simulink model "PMSM_FOC_Traction"  (R2020b)
settings: Solver=FixedStepAuto  StartTime=0.0  StopTime=10  RelTol=1e-3
model workspace (MAT data in the model file):
  wc : Simulink.Parameter (value not decoded)
values from neighbouring files (symbols this model uses):
  Cosine_table = 1.0 0.99999529 0.99999058 0.99998587 0.99998116 0.99996704 0.99995291 0.99993885 0.99992472 0.99990118 0.99987763 0.99985409 0.9998306 0.99979764 0.99976468 0.99973178 0.99969882 0.99965644 0.99961412 0.99957174 0.99952942 0.99947762 0.99942589 0.99937415 0.99932235 0.9992612 0.99920005 0.99913889 0.99907768 0.99900717 0.99893659 0.99886602 0.99879545 0.99871546 0.99863547 0.99855554 0.99847555 0.    [Hall_HSMO_FOC_Data.sldd]    (also in Hall_SMO_FOC_Data.sldd)
  Flux = 0.0109    [G474_FOC_HSMO.sldd]    (also in Hall_HSMO_FOC_Data.sldd = 0.00529276
  MTPA_id_table = 0.22889 0.23462678 0.23770036 0.2381243 0.23591207 0.23107713 0.2236329 0.21359272 0.20096992 0.18577772 0.16802935 0.14773798 0.12491672 0.099578641 0.071736768 0.041404068 0.0085934745 -0.026682133 -0.064409919 -0.10457709 -0.14717092 -0.1921787 -0.2395878 -0.28938559 -0.34155953 -0.39609709 -0.45298585 -0.51221335 -0.57376724 -0.63763517 -0.70380485 -0.77226412 -0.84300071 -0.91600245 -0.991257    [Hall_HSMO_FOC_Data.sldd]    (also in Hall_SMO_FOC_Data.sldd)
  MTPA_iq_table = -1.0417 -0.16083497 0.71926296 1.5985928 2.4771533 3.3549435 4.2319627 5.1082091 5.9836826 6.8583813 7.732305 8.6054525 9.4778223 10.349415 11.220228 12.090261 12.959513 13.827983 14.69567 15.562573 16.428694 17.294027 18.158575 19.022335 19.885307 20.747492 21.608887 22.469492 23.329306 24.188328 25.046556 25.903992 26.760633 27.616482 28.471533 29.325788 30.179247 31.031908 31.883772 32.734837 3    [Hall_HSMO_FOC_Data.sldd]    (also in Hall_SMO_FOC_Data.sldd)
  MTPA_Te_Max = 800.0    [Hall_HSMO_FOC_Data.sldd]    (also in Hall_SMO_FOC_Data.sldd)
  MTPA_Te_Min = 0.0    [Hall_HSMO_FOC_Data.sldd]    (also in Hall_SMO_FOC_Data.sldd)
  Sine_table = 0.0 0.0015339879 0.0030679768 0.0046019657 0.0061359555 0.0076698866 0.0092038177 0.010737749 0.012271681 0.013805497 0.015339312 0.016873131 0.018406944 0.019940587 0.021474229 0.023007872 0.024541514 0.026074925 0.027608337 0.029141748 0.03067516 0.032208283 0.033741407 0.035274528 0.036807653 0.038340431 0.039873205 0.04140598 0.042938754 0.04447113 0.046003502 0.047535874 0.049068246 0.0506001    [Hall_HSMO_FOC_Data.sldd]    (also in Hall_SMO_FOC_Data.sldd)
undefined symbols (not defined in the file or in its folder): CL_Param, ctrlParamsPI, DiscIntNeverNeededParam, Flux_weak, FluxObsever, Hall_Parameter, HFI, inverter, Kiv, Kiw, Kpv, Kpw, magnitude, OPL_Param, pmsm, Resolver_Parameter, sigbuilder_block, SMO, SVPWM, Vdc
libraries: powerlib x29, fl_lib x18, simulink x7, nesl_utility x7, pid_lib x5, dspstat3 x4, eeGeneralControl x4, eeDiscretePi x2, powerlib_extras x1, ee_lib x1
(part 5 of 6)

== system PMSM_FOC_Traction/Motor_Control/Motor_Control_Funtion/Control_Command_2ms/Speed_PI/Speed_PI/Speed_Control ==
  Err : Inport
  Action Port : ActionPort  ActionPortLabel=if((u1==3)&(u2==1))
  Add : Sum
  Cons : Constant  Value=0  OutDataTypeStr=single
  Discrete-Time Integrator : DiscreteIntegrator  SampleTime=-1  ICPrevOutput=DiscIntNeverNeededParam  ICPrevScaledInput=DiscIntNeverNeededParam
  Ki : Constant  Value=ctrlParamsPI.speed_PI_Ki  OutDataTypeStr=single
  Kp : Constant  Value=ctrlParamsPI.speed_PI_Kp  OutDataTypeStr=single
  Product : Product
  Product1 : Product
  Relational Operator1 : RelationalOperator  Operator===  OutDataTypeStr=boolean  RndMeth=Simplest
  Saturation : Saturate  UpperLimit=ctrlParamsPI.speed_PI_OutputMax  LowerLimit=ctrlParamsPI.speed_PI_OutputMin
  Scope : Scope
  Switch : Switch  Criteria=u2 > Threshold
  Unit Delay3 : UnitDelay  SampleTime=-1  HasFrameUpgradeWarning=on
  PI_Out : Outport
  wires:
  Kp/1 -> Product/1
  Err/1 -> Switch/1, Product/2
  Switch/1 -> Product1/2
  Product1/1 -> Discrete-Time Integrator/1
  Product/1 -> Add/1
  Add/1 -> Relational Operator1/1, Saturation/1
  Saturation/1 -> Relational Operator1/2, PI_Out/1
  Discrete-Time Integrator/1 -> Add/2, Scope/1
  Relational Operator1/1 -> Unit Delay3/1
  Ki/1 -> Product1/1
  Unit Delay3/1 -> Switch/2
  Cons/1 -> Switch/3

== system PMSM_FOC_Traction/Motor_Control/Motor_Control_Funtion/Control_Command_2ms/Speed_PI/Speed_PI/Speed_Control1 ==
  Err : Inport
  Action Port : ActionPort  ActionPortLabel=elseif((u2==0) & ((u3~=2)&(u3~=3)))
  Add : Sum
  Cons : Constant  Value=0  OutDataTypeStr=single
  Discrete-Time Integrator : DiscreteIntegrator  SampleTime=-1  ICPrevOutput=DiscIntNeverNeededParam  ICPrevScaledInput=DiscIntNeverNeededParam
  Ki : Constant  Value=ctrlParamsPI.speed_PI_Ki  OutDataTypeStr=single
  Kp : Constant  Value=ctrlParamsPI.speed_PI_Kp  OutDataTypeStr=single
  Product : Product
  Product1 : Product
  Relational Operator1 : RelationalOperator  Operator===  OutDataTypeStr=boolean  RndMeth=Simplest
  Saturation : Saturate  UpperLimit=ctrlParamsPI.speed_PI_OutputMax  LowerLimit=ctrlParamsPI.speed_PI_OutputMin
  Switch : Switch  Criteria=u2 > Threshold
  Unit Delay3 : UnitDelay  SampleTime=-1  HasFrameUpgradeWarning=on
  PI_Out : Outport
  wires:
  Kp/1 -> Product/1
  Err/1 -> Switch/1, Product/2
  Switch/1 -> Product1/2
  Product1/1 -> Discrete-Time Integrator/1
  Product/1 -> Add/1
  Add/1 -> Relational Operator1/1, Saturation/1
  Saturation/1 -> Relational Operator1/2, PI_Out/1
  Discrete-Time Integrator/1 -> Add/2
  Relational Operator1/1 -> Unit Delay3/1
  Ki/1 -> Product1/1
  Unit Delay3/1 -> Switch/2
  Cons/1 -> Switch/3

== system PMSM_FOC_Traction/Motor_Control/Motor_Control_Funtion/FOC_Control_100us/FOC/Angle_set/Subsystem ==
  HFI_state : Inport
  HFI_angle : Inport  Port=2
  IPD_Angle : Inport  Port=3
  Action Port : ActionPort  ActionPortLabel=if(u1 ==1)
  If1 : If  IfExpression=u1 ==3  ElseIfExpressions=u1 <3  ShowElse=off
  Merge : Merge
  Subsystem1 : Subsystem
  Subsystem2 : Subsystem
  Out1 : Outport
  wires:
  HFI_state/1 -> If1/1
  HFI_angle/1 -> Subsystem1/1(HFI_Angle)
  If1/2 -> Subsystem2/Action
  If1/1 -> Subsystem1/Action
  IPD_Angle/1 -> Subsystem2/1(IPD_Angle)
  Merge/1 -> Out1/1
  Subsystem1/1(Out1) -> Merge/1
  Subsystem2/1(Out1) -> Merge/2

== system PMSM_FOC_Traction/Motor_Control/Motor_Control_Funtion/FOC_Control_100us/FOC/Angle_set/Subsystem1 ==
  Reso_angle : Inport
  Action Port : ActionPort  ActionPortLabel=else
  Out1 : Outport
  wires:
  Reso_angle/1 -> Out1/1

== system PMSM_FOC_Traction/Motor_Control/Motor_Control_Funtion/FOC_Control_100us/FOC/Clarke_Transform/Clark1 ==
  Iabc : Inport
  Add : Sum  Inputs=+--
  Add1 : Sum  Inputs=+-
  Demux : Demux  Outputs=3
  Gain : Gain  Gain=0.5
  Gain1 : Gain  Gain=0.5
  Gain2 : Gain  Gain=sqrt(2/3)
  Gain3 : Gain  Gain=sqrt(3)/2
  Gain4 : Gain  Gain=sqrt(3)/2
  Gain5 : Gain  Gain=sqrt(2/3)
  Ialpha : Outport  VectorParamsAs1DForOutWhenUnconnected=off
  Ibeta : Outport  Port=2  VectorParamsAs1DForOutWhenUnconnected=off
  wires:
  Iabc/1 -> Demux/1
  Demux/1 -> Add/1
  Gain/1 -> Add/2
  Demux/2 -> Gain3/1, Gain/1
  Gain1/1 -> Add/3
  Demux/3 -> Gain4/1, Gain1/1
  Add/1 -> Gain2/1
  Gain2/1 -> Ialpha/1
  Gain3/1 -> Add1/1
  Gain4/1 -> Add1/2
  Add1/1 -> Gain5/1
  Gain5/1 -> Ibeta/1

== system PMSM_FOC_Traction/Motor_Control/Motor_Control_Funtion/FOC_Control_100us/FOC/D_Current_PI/ID_Control ==
  Err : Inport
  Add : Sum
  Cons : Constant  Value=0  OutDataTypeStr=single
  Discrete-Time Integrator : DiscreteIntegrator  SampleTime=-1  ICPrevOutput=DiscIntNeverNeededParam  ICPrevScaledInput=DiscIntNeverNeededParam
  Ki : Constant  Value=ctrlParamsPI.ID_Current_PI_Ki  OutDataTypeStr=single
  Kp : Constant  Value=ctrlParamsPI.ID_Current_PI_Kp  OutDataTypeStr=single
  Product : Product
  Product1 : Product
  Relational Operator1 : RelationalOperator  Operator===  OutDataTypeStr=boolean  RndMeth=Simplest
  Saturation : Saturate  UpperLimit=ctrlParamsPI.ID_Current_PI_OutputMax  LowerLimit=ctrlParamsPI.ID_Current_PI_OutputMin
  Switch : Switch  Criteria=u2 > Threshold
  Unit Delay3 : UnitDelay  SampleTime=-1  HasFrameUpgradeWarning=on
  PI_Out : Outport
  wires:
  Kp/1 -> Product/1
  Err/1 -> Switch/1, Product/2
  Switch/1 -> Product1/2
  Product1/1 -> Discrete-Time Integrator/1
  Product/1 -> Add/1
  Add/1 -> Relational Operator1/1, Saturation/1
  Saturation/1 -> Relational Operator1/2, PI_Out/1
  Cons/1 -> Switch/3
  Discrete-Time Integrator/1 -> Add/2
  Relational Operator1/1 -> Unit Delay3/1
  Ki/1 -> Product1/1
  Unit Delay3/1 -> Switch/2

== system PMSM_FOC_Traction/Motor_Control/Motor_Control_Funtion/FOC_Control_100us/FOC/Flux_weakening /Subsystem ==
  Vd : Inport
  Vq : Inport  Port=2
  Id : Inport  Port=3
  Iq : Inport  Port=4
  Action Port : ActionPort  ActionPortLabel=if(u1 ==1)
  Flux_weak : Subsystem  TreatAsAtomicUnit=on  mask{kp=Flux_weak.Kp, ki=Flux_weak.Ki, Id_max=Flux_weak.Idref_max, Id_min=Flux_weak.Idref_min}
      settings: RTWSystemCode=Nonreusable function  RTWFcnNameOpts=Use subsystem name
  Id_ref : Outport
  Iq_ref : Outport  Port=2
  wires:
  Vd/1 -> Flux_weak/1(Vd)
  Vq/1 -> Flux_weak/2(Vq)
  Id/1 -> Flux_weak/3(id_input)
  Iq/1 -> Flux_weak/4(Iq_input)
  Flux_weak/1(Id_ref) -> Id_ref/1
  Flux_weak/2(iq_ref) -> Iq_ref/1

== system PMSM_FOC_Traction/Motor_Control/Motor_Control_Funtion/FOC_Control_100us/FOC/Flux_weakening /Subsystem1 ==
  Id : Inport
  Iq : Inport  Port=2
  Action Port : ActionPort  ActionPortLabel=else
  Id_ref : Outport
  Iq_ref : Outport  Port=2
  wires:
  Id/1 -> Id_ref/1
  Iq/1 -> Iq_ref/1

== system PMSM_FOC_Traction/Motor_Control/Motor_Control_Funtion/FOC_Control_100us/FOC/HF_Observer/HFI_Function ==
  Ialpha-beta : Inport
  Phase_CurrentABC : Inport  Port=2  PortDimensions=3
  Id : Inport  Port=3
  Action Port : ActionPort  ActionPortLabel=if(u1==1)
  Delay : Delay  DelayLength=1  InitialCondition=0
  Delay1 : Delay  DelayLength=1  InitialCondition=0
  Delay2 : Delay  DelayLength=1  InitialCondition=0
  HFI : Subsystem
  HFI_Enalble : Constant  Value=HFI.Func_Enable  OutDataTypeStr=uint8
  HFI_State_machine : Stateflow chart  TreatAsAtomicUnit=on
      settings: RTWSystemCode=Nonreusable function  RTWFcnNameOpts=Use subsystem name
  IPD : Subsystem  TreatAsAtomicUnit=on
      settings: RTWSystemCode=Nonreusable function
  Merge : Merge
  Merge1 : Merge
  Merge2 : Merge
  NS : Subsystem  TreatAsAtomicUnit=on
      settings: RTWSystemCode=Nonreusable function
  Switch Case1 : SwitchCase  CaseConditions={1,2,3}
  RUN_State : Outport
  HFI_State : Outport  Port=2
  HFI_signal : Outport  Port=3
  speed_est : Outport  Port=4
  theta_est : Outport  Port=5
  Ualpha : Outport  Port=6
  Ubeta : Outport  Port=7
  IPD_Theta : Outport  Port=8
  wires:
  NS/1(Ualpha) -> Merge/2
  HFI_State_machine/1(HFI_state) -> HFI_State/1, Switch Case1/1
  Delay/1 -> NS/1(Id)
  Switch Case1/2 -> [NS]
  Id/1 -> Delay/1
  IPD/2(Ubeta) -> Merge1/1
  [NS] -> NS/Action
  HFI/5(theta_est) -> Merge2/2
  IPD/3(Theta) -> Delay1/1
  Phase_CurrentABC/1 -> IPD/1(Iabc)  "Phase_CurrentABC"
  Delay1/1 -> NS/2(Theta)
  HFI/2(speed_est) -> speed_est/1
  Ialpha-beta/1 -> HFI/1(Ialpha-beta)
  Merge1/1 -> Ubeta/1
  Switch Case1/4 -> [default]
  [IPD] -> IPD/Action
  Merge/1 -> Ualpha/1
  [RUN] -> HFI/Action
  NS/2(Ubeta) -> Merge1/2
  Switch Case1/1 -> [IPD]
  HFI_Enalble/1 -> HFI_State_machine/1(HFI_flag)
  HFI/1(HFI_signal) -> HFI_signal/1
  IPD/1(Ualpha) -> Merge/1
  NS/3(IPD_Angle) -> Merge2/1
  Merge2/1 -> theta_est/1
  Switch Case1/3 -> [RUN]
  NS/4(Angle_RUN) -> Delay2/1
  Delay2/1 -> HFI/2(IPD_angle)
  HFI/3(HFI_State) -> RUN_State/1
  HFI/4(IPD_Theta) -> IPD_Theta/1

== system PMSM_FOC_Traction/Motor_Control/Motor_Control_Funtion/FOC_Control_100us/FOC/Q_Current_PI/IQ_Control ==
  Err : Inport
  Add : Sum
  Cons : Constant  Value=0  OutDataTypeStr=single
  Discrete-Time Integrator : DiscreteIntegrator  SampleTime=-1  ICPrevOutput=DiscIntNeverNeededParam  ICPrevScaledInput=DiscIntNeverNeededParam
  Ki : Constant  Value=ctrlParamsPI.IQ_Current_PI_Ki  OutDataTypeStr=single
  Kp : Constant  Value=ctrlParamsPI.IQ_Current_PI_Kp  OutDataTypeStr=single
  Product : Product
  Product1 : Product
  Relational Operator1 : RelationalOperator  Operator===  OutDataTypeStr=boolean  RndMeth=Simplest
  Saturation : Saturate  UpperLimit=ctrlParamsPI.IQ_Current_PI_OutputMax  LowerLimit=ctrlParamsPI.IQ_Current_PI_OutputMin
  Switch : Switch  Criteria=u2 > Threshold
  Unit Delay3 : UnitDelay  SampleTime=-1  HasFrameUpgradeWarning=on
  PI_Out : Outport
  wires:
  Kp/1 -> Product/1
  Err/1 -> Switch/1, Product/2
  Switch/1 -> Product1/2
  Product1/1 -> Discrete-Time Integrator/1
  Product/1 -> Add/1
  Add/1 -> Relational Operator1/1, Saturation/1
  Saturation/1 -> Relational Operator1/2, PI_Out/1
  Cons/1 -> Switch/3
  Discrete-Time Integrator/1 -> Add/2
  Relational Operator1/1 -> Unit Delay3/1
  Ki/1 -> Product1/1
  Unit Delay3/1 -> Switch/2

== system PMSM_FOC_Traction/Motor_Control/Motor_Control_Funtion/FOC_Control_100us/FOC/SVPWM/N Sector  Caculate ==
  Ubelta : Inport
  Ualf : Inport  Port=2
  Add : Sum  Inputs=+++
  Add1 : Sum  Inputs=-+
  Add2 : Sum  Inputs=--
  Constant : Constant  OutDataTypeStr=single
  Constant1 : Constant  Value=0  OutDataTypeStr=single
  Gain : Gain  Gain=sqrt(3)
  Gain1 : Gain  Gain=2
  Gain2 : Gain  Gain=4
  Saturation : Saturate  UpperLimit=6  LowerLimit=1
  Switch : Switch
  Switch1 : Switch
  Switch2 : Switch
  N : Outport
  wires:
  Saturation/1 -> N/1
  Add/1 -> Saturation/1
  Gain2/1 -> Add/3
  Switch2/1 -> Gain2/1
  Add2/1 -> Switch2/2
  Gain1/1 -> Add/2
  Switch1/1 -> Gain1/1
  Add1/1 -> Switch1/2
  Gain/1 -> Add2/2, Add1/2
  Ualf/1 -> Gain/1
  Switch/1 -> Add/1
  Constant1/1 -> Switch/3, Switch1/3, Switch2/3
  Constant/1 -> Switch/1, Switch1/1, Switch2/1
  Ubelta/1 -> Add2/1, Add1/1, Switch/2

== system PMSM_FOC_Traction/Motor_Control/Motor_Control_Funtion/FOC_Control_100us/FOC/SVPWM/T1 T2  Caculate ==
  note: Z
  note: Y
  note: -X
  note: X
  note: -Y
  note: Y
  note: -X
  note: X
  note: Z
  note: -Y
  note: -Z
  note: X
  note: Y
  note: Z
  N : Inport
  X : Inport  Port=2
  Y : Inport  Port=3
  Z : Inport  Port=4
  Tpwm : Inport  Port=5
  Add : Sum
  Add1 : Sum  Inputs=-+
  Divide : Product  Inputs=**/
  Divide1 : Product  Inputs=/**
  Gain : Gain  Gain=-1
  Gain1 : Gain  Gain=-1
  Gain2 : Gain  Gain=-1
  Index Vector : MultiPortSwitch  Inputs=6
  Index Vector1 : MultiPortSwitch  Inputs=6
  Switch : Switch  Criteria=u2 > Threshold
  Switch2 : Switch  Criteria=u2 > Threshold
  T1 : Outport
  T2 : Outport  Port=2
  wires:
  Switch2/1 -> T2/1
  Divide1/1 -> Switch2/3
  Switch/1 -> T1/1
  Add1/1 -> Switch/2, Switch2/2
  Add/1 -> Divide1/1, Divide/3, Add1/1
  Tpwm/1 -> Divide1/2, Divide/2, Add1/2
  Divide/1 -> Switch/3
  Index Vector1/1 -> Switch2/1, Add/2, Divide1/3
  Index Vector/1 -> Switch/1, Divide/1, Add/1
  Gain1/1 -> Index Vector/7, Index Vector1/6
  Gain2/1 -> Index Vector/4, Index Vector1/7  "-Z"
  Gain/1 -> Index Vector/5, Index Vector1/3
  Y/1 -> Gain1/1, Index Vector/3, Index Vector1/2
  X/1 -> Index Vector1/4, Index Vector/6, Gain/1
  Z/1 -> Index Vector/2, Index Vector1/5, Gain2/1
  N/1 -> Index Vector1/1, Index Vector/1

== system PMSM_FOC_Traction/Motor_Control/Motor_Control_Funtion/FOC_Control_100us/FOC/SVPWM/Tcm calculate ==
  note: Tc
  note: Tb
  note: Ta
  N : Inport
  T1 : Inport  Port=2
  T2 : Inport  Port=3
  Tpwm : Inport  Port=4
  Add : Sum  Inputs=--+
  Add1 : Sum
  Add2 : Sum
  Gain : Gain  Gain=0.5
  Gain1 : Gain  Gain=0.5
  Gain2 : Gain  Gain=1/4
  Index Vector : MultiPortSwitch  Inputs=6
  Index Vector1 : MultiPortSwitch  Inputs=6
  Index Vector2 : MultiPortSwitch  Inputs=6
  Scope2 : Scope  NumInputPorts=3
  Tcm1 : Outport
  Tcm2 : Outport  Port=2
  Tcm3 : Outport  Port=3
  wires:
  Index Vector2/1 -> Scope2/3, Tcm3/1
  N/1 -> Index Vector/1, Index Vector1/1, Index Vector2/1
  Add2/1 -> Index Vector/5, Index Vector/6, Index Vector1/3, Index Vector1/7, Index Vector2/2, Index Vector2/4
  Gain1/1 -> Add2/1
  Add1/1 -> Add2/2, Index Vector/2, Index Vector/7, Index Vector1/4, Index Vector1/5, Index Vector2/3, Index Vector2/6
  Gain2/1 -> Index Vector2/5, Index Vector2/7, Add1/2, Index Vector/3, Index Vector/4, Index Vector1/2, Index Vector1/6
  Gain/1 -> Add1/1
  Add/1 -> Gain2/1
  Tpwm/1 -> Add/3
  T2/1 -> Add/2, Gain1/1
  T1/1 -> Add/1, Gain/1
  Index Vector/1 -> Scope2/1, Tcm1/1
  Index Vector1/1 -> Scope2/2, Tcm2/1

== system PMSM_FOC_Traction/Motor_Control/Motor_Control_Funtion/FOC_Control_100us/FOC/SVPWM/XYZ Caculate ==
  note: X
  note: Y
  note: Z
  Ualfpa : Inport
  Ubelta : Inport  Port=2
  Udc : Inport  Port=3
  Tpwm : Inport  Port=4
  Add1 : Sum  Inputs=-+
  Add2 : Sum  Inputs=--
  Constant : Constant  Value=sqrt(3)  OutDataTypeStr=single
  Divide : Product  Inputs=**/
  Gain : Gain  Gain=sqrt(3)
  Gain1 : Gain  Gain=-0.5
  Gain2 : Gain  Gain=-0.5
  Product : Product
  Product1 : Product
  Product2 : Product
  X : Outport
  Y : Outport  Port=2
  Z : Outport  Port=3
  wires:
  Gain2/1 -> Product1/1
  Add2/1 -> Gain2/1
  Add1/1 -> Gain1/1
  Gain/1 -> Add2/2, Add1/2
  Ualfpa/1 -> Gain/1
  Ubelta/1 -> Add2/1, Add1/1, Product/1
  Gain1/1 -> Product2/2
  Product2/1 -> Z/1
  Divide/1 -> Product1/2, Product2/1, Product/2
  Product1/1 -> Y/1
  Product/1 -> X/1
  Udc/1 -> Divide/3
  Tpwm/1 -> Divide/2
  Constant/1 -> Divide/1

== system PMSM_FOC_Traction/Motor_Control/Motor_Control_Funtion/FOC_Control_100us/FOC/Set_Idq/Set_Idq ==
  Id_Command : Inport
  Iq_Command : Inport  Port=2
  Action Port : ActionPort  ActionPortLabel=if(u1==2 | u1==1)
  Id : Outport  VectorParamsAs1DForOutWhenUnconnected=off
  Iq : Outport  Port=2  VectorParamsAs1DForOutWhenUnconnected=off
  wires:
  Id_Command/1 -> Id/1
  Iq_Command/1 -> Iq/1

== system PMSM_FOC_Traction/Motor_Control/Motor_Control_Funtion/FOC_Control_100us/FOC/Set_Idq/Set_Idq1 ==
  Id_Command : Inport
  Iq_Command : Inport  Port=2
  Action Port : ActionPort  ActionPortLabel=else
  Id : Outport  VectorParamsAs1DForOutWhenUnconnected=off
  Iq : Outport  Port=2  VectorParamsAs1DForOutWhenUnconnected=off
  wires:
  Id_Command/1 -> Id/1
  Iq_Command/1 -> Iq/1

== system PMSM_FOC_Traction/Motor_Control/Motor_Control_Funtion/FOC_Control_100us/FOC/Subsystem1/If Action Subsystem1 ==
  In1 : Inport
  In2 : Inport  Port=2
  Action Port : ActionPort  ActionPortLabel=else
  Out1 : Outport
  Out2 : Outport  Port=2
  wires:
  In1/1 -> Out1/1
  In2/1 -> Out2/1

== system PMSM_FOC_Traction/Motor_Control/Motor_Control_Funtion/FOC_Control_100us/FOC/Subsystem1/If Action Subsystem2 ==
  In1 : Inport
  In2 : Inport  Port=2
  Action Port : ActionPort  ActionPortLabel=if((u1<3)&(u1>0))
  Out1 : Outport
  Out2 : Outport  Port=2
  wires:
  In1/1 -> Out1/1
  In2/1 -> Out2/1

== system PMSM_FOC_Traction/Motor_Control/Motor_Control_Funtion/Angle_Speed_100us/Flux_OBSERVER/equ3.12/integrator/RangeLimit ==
  In : Inport  OutDataTypeStr=single
  Constant : Constant  Value=2*pi  OutDataTypeStr=single  SampleTime=-1
  Constant1 : Constant  Value=0  OutDataTypeStr=single  SampleTime=-1
  If : If  NumInputs=2  IfExpression=u1  ElseIfExpressions=u2
  If Action Subsystem : Subsystem  TreatAsAtomicUnit=on
  If Action Subsystem1 : Subsystem  TreatAsAtomicUnit=on
  If Action Subsystem2 : Subsystem  TreatAsAtomicUnit=on
  Merge : Merge  Inputs=3
  Relational Operator : RelationalOperator  Operator=>  OutDataTypeStr=boolean  RndMeth=Simplest
  Relational Operator1 : RelationalOperator  Operator=<  OutDataTypeStr=boolean  RndMeth=Simplest
  Theta : Outport  OutDataTypeStr=single
  wires:
  Relational Operator/1 -> If/1
  Constant/1 -> Relational Operator/2
  Constant1/1 -> Relational Operator1/2
  In/1 -> Relational Operator1/1, If Action Subsystem2/1(In1), If Action Subsystem1/1(In1), If Action Subsystem/1(In1), Relational Operator/1
  Relational Operator1/1 -> If/2
  Merge/1 -> Theta/1
  If/3 -> If Action Subsystem2/Action
  If/2 -> If Action Subsystem/Action
  If/1 -> If Action Subsystem1/Action
  If Action Subsystem2/1(Out1) -> Merge/1
  If Action Subsystem/1(Out1) -> Merge/2
  If Action Subsystem1/1(Out1) -> Merge/3

== system PMSM_FOC_Traction/Motor_Control/Motor_Control_Funtion/Angle_Speed_100us/HIGH_SMO/QPLL/SpeedToTheta/RangeLimit ==
  In : Inport
  Constant : Constant  Value=2*pi  OutDataTypeStr=single  SampleTime=-1
  Constant1 : Constant  Value=0  OutDataTypeStr=single  SampleTime=-1
  If : If  NumInputs=2  IfExpression=u1  ElseIfExpressions=u2
  If Action Subsystem : Subsystem  TreatAsAtomicUnit=on
  If Action Subsystem1 : Subsystem  TreatAsAtomicUnit=on
  If Action Subsystem2 : Subsystem  TreatAsAtomicUnit=on
  Merge : Merge  Inputs=3
  Relational Operator : RelationalOperator  Operator=>  OutDataTypeStr=boolean  RndMeth=Simplest
  Relational Operator1 : RelationalOperator  Operator=<  OutDataTypeStr=boolean  RndMeth=Simplest
  Theta : Outport
  wires:
  Relational Operator/1 -> If/1
  Constant/1 -> Relational Operator/2
  Constant1/1 -> Relational Operator1/2
  In/1 -> Relational Operator1/1, If Action Subsystem2/1(In1), If Action Subsystem1/1(In1), If Action Subsystem/1(In1), Relational Operator/1
  Relational Operator1/1 -> If/2
  Merge/1 -> Theta/1
  If/3 -> If Action Subsystem2/Action
  If/2 -> If Action Subsystem/Action
  If/1 -> If Action Subsystem1/Action
  If Action Subsystem2/1(Out1) -> Merge/1
  If Action Subsystem/1(Out1) -> Merge/2
  If Action Subsystem1/1(Out1) -> Merge/3

== system PMSM_FOC_Traction/Motor_Control/Motor_Control_Funtion/Angle_Speed_100us/HIGH_SMO/QPLL/Subsystem1/If Action Subsystem ==
  Action Port : ActionPort  ActionPortLabel=if(u1 > 0)
  Constant : Constant  OutDataTypeStr=single
  Out1 : Outport
  wires:
  Constant/1 -> Out1/1

== system PMSM_FOC_Traction/Motor_Control/Motor_Control_Funtion/Angle_Speed_100us/HIGH_SMO/QPLL/Subsystem1/If Action Subsystem1 ==
  Action Port : ActionPort  ActionPortLabel=else
  Constant : Constant  Value=-1  OutDataTypeStr=single
  Out1 : Outport
  wires:
  Constant/1 -> Out1/1

== system PMSM_FOC_Traction/Motor_Control/Motor_Control_Funtion/Angle_Speed_100us/SpeedAndAngle/ACC_OMG/BLDC/Control ==
  RPMReq : Inport
  w_sens : Inport  Port=2
  Hall : Inport  Port=3
  BLDC_State : Inport  Port=4
  Commutation : Subsystem
  If1 : If  IfExpression=u1==3  ShowElse=off
  Scope3 : Scope
  Speed_Control : Subsystem
  Sum : Sum  Inputs=|+-
  rad/s->rpm : Gain  Gain=30/pi
  Gate : Outport  VectorParamsAs1DForOutWhenUnconnected=off
  Duty : Outport  Port=2  VectorParamsAs1DForOutWhenUnconnected=off
  wires:
  RPMReq/1 -> Sum/1
  w_sens/1 -> rad/s->rpm/1
  rad/s->rpm/1 -> Sum/2, Scope3/1
  Commutation/1(S) -> Gate/1
  Hall/1 -> Commutation/1(Hall)
  Sum/1 -> Speed_Control/1(Err)
  Speed_Control/1(PI_Out) -> Duty/1
  BLDC_State/1 -> If1/1
  If1/1 -> Speed_Control/Action

== system PMSM_FOC_Traction/Motor_Control/Motor_Control_Funtion/Angle_Speed_100us/SpeedAndAngle/ACC_OMG/Six_point/Sector_1 ==
  Action Port : ActionPort  ActionPortLabel=case [ 1 ]:
  Add : Sum
  Constant : Constant  Value=Hall_Parameter.Sector_1  OutDataTypeStr=single
  Constant1 : Constant  Value=Hall_Parameter.shift  OutDataTypeStr=single
  Angle_0 : Outport
  wires:
  Constant/1 -> Add/1
  Constant1/1 -> Add/2
  Add/1 -> Angle_0/1

== system PMSM_FOC_Traction/Motor_Control/Motor_Control_Funtion/Angle_Speed_100us/SpeedAndAngle/ACC_OMG/Six_point/Sector_2 ==
  Action Port : ActionPort  ActionPortLabel=case [ 2 ]:
  Add : Sum
  Constant1 : Constant  Value=Hall_Parameter.shift  OutDataTypeStr=single
  Pi/3 : Constant  Value=Hall_Parameter.Sector_2  OutDataTypeStr=single
  Angle_0 : Outport
  wires:
  Pi/3/1 -> Add/1
  Constant1/1 -> Add/2
  Add/1 -> Angle_0/1

== system PMSM_FOC_Traction/Motor_Control/Motor_Control_Funtion/Angle_Speed_100us/SpeedAndAngle/ACC_OMG/Six_point/Sector_3 ==
  Action Port : ActionPort  ActionPortLabel=case [ 3 ]:
  Add : Sum
  Constant : Constant  Value=Hall_Parameter.Sector_3  OutDataTypeStr=single
  Constant1 : Constant  Value=Hall_Parameter.shift  OutDataTypeStr=single
  Angle_0 : Outport
  wires:
  Constant/1 -> Add/1
  Add/1 -> Angle_0/1
  Constant1/1 -> Add/2

== system PMSM_FOC_Traction/Motor_Control/Motor_Control_Funtion/Angle_Speed_100us/SpeedAndAngle/ACC_OMG/Six_point/Sector_4 ==
  Action Port : ActionPort  ActionPortLabel=case [ 4 ]:
  Add : Sum
  Constant : Constant  Value=Hall_Parameter.Sector_4  OutDataTypeStr=single
  Constant1 : Constant  Value=Hall_Parameter.shift  OutDataTypeStr=single
  Angle_0 : Outport
  wires:
  Constant/1 -> Add/1
  Add/1 -> Angle_0/1
  Constant1/1 -> Add/2

== system PMSM_FOC_Traction/Motor_Control/Motor_Control_Funtion/Angle_Speed_100us/SpeedAndAngle/ACC_OMG/Six_point/Sector_5 ==
  Action Port : ActionPort  ActionPortLabel=case [ 5 ]:
  Add : Sum
  Constant : Constant  Value=Hall_Parameter.Sector_5  OutDataTypeStr=single
  Constant1 : Constant  Value=Hall_Parameter.shift  OutDataTypeStr=single
  Angle_0 : Outport
  wires:
  Constant/1 -> Add/1
  Add/1 -> Angle_0/1
  Constant1/1 -> Add/2

== system PMSM_FOC_Traction/Motor_Control/Motor_Control_Funtion/Angle_Speed_100us/SpeedAndAngle/ACC_OMG/Six_point/Sector_6 ==
  Action Port : ActionPort  ActionPortLabel=case [ 6 ]:
  Add : Sum
  Constant : Constant  Value=Hall_Parameter.Sector_6  OutDataTypeStr=single
  Constant1 : Constant  Value=Hall_Parameter.shift  OutDataTypeStr=single
  Angle_0 : Outport
  wires:
  Constant/1 -> Add/1
  Add/1 -> Angle_0/1
  Constant1/1 -> Add/2

== system PMSM_FOC_Traction/Motor_Control/Motor_Control_Funtion/Angle_Speed_100us/SpeedAndAngle/ADC_IRQ/HallAngle_calibration/If Action Subsystem1 ==
  In1 : Inport
  Action Port : ActionPort  ActionPortLabel=else
  Out1 : Outport
  wires:
  In1/1 -> Out1/1

== system PMSM_FOC_Traction/Motor_Control/Motor_Control_Funtion/Angle_Speed_100us/SpeedAndAngle/ADC_IRQ/HallAngle_calibration/If Action Subsystem2 ==
  In1 : Inport
  Action Port : ActionPort  ActionPortLabel=if(u1 > 6.283185307)
  2pi : Constant  Value=2*pi  OutDataTypeStr=single
  Subtract1 : Sum  Inputs=+-  OutDataTypeStr=single
  Out1 : Outport
  wires:
  In1/1 -> Subtract1/1
  Subtract1/1 -> Out1/1
  2pi/1 -> Subtract1/2

== system PMSM_FOC_Traction/Motor_Control/Motor_Control_Funtion/Angle_Speed_100us/SpeedAndAngle/ADC_IRQ/HallAngle_calibration/If Action Subsystem3 ==
  In1 : Inport
  Action Port : ActionPort  ActionPortLabel=elseif(u1<0)
  Angle_offset : Constant  Value=2*pi  OutDataTypeStr=single
  Subtract1 : Sum
  Out1 : Outport
  wires:
  In1/1 -> Subtract1/1
  Subtract1/1 -> Out1/1
  Angle_offset/1 -> Subtract1/2

== system PMSM_FOC_Traction/Motor_Control/Motor_Control_Funtion/Angle_Speed_100us/SpeedAndAngle/Subsystem/Subsystem/Commutation ==
  Constant : Constant  OutDataTypeStr=uint8
  Direct Lookup Table (n-D)2 : LookupNDDirect  InputsSelectThisObjectFromTable=Vector  Table=[0 0 0 1 1 0;0 1 1 0 0 0;0 1 0 0 0 1;1 0 0 0 1 0;1 0 1 0 0 0;0 0 0 1 0 1]  TableDataTypeStr=single
  Scope : Scope
  S : Outport  VectorParamsAs1DForOutWhenUnconnected=off
  wires:
  Direct Lookup Table (n-D)2/1 -> S/1
  Constant/1 -> Scope/1, Direct Lookup Table (n-D)2/1

== system PMSM_FOC_Traction/Motor_Control/Motor_Control_Funtion/Angle_Speed_100us/SpeedAndAngle/Subsystem/Subsystem1/Commutation ==
  Hall : Inport
  Bias : Bias  Bias=-1
  Bit concatenate : Subsystem
  Data Type Conversion : DataTypeConversion
  Direct Lookup Table (n-D)2 : LookupNDDirect  InputsSelectThisObjectFromTable=Vector  Table=[0 0 0 1 1 0;0 1 1 0 0 0;0 1 0 0 0 1;1 0 0 0 1 0;1 0 1 0 0 0;0 0 0 1 0 1]  TableDataTypeStr=single
  Scope : Scope
  S : Outport  VectorParamsAs1DForOutWhenUnconnected=off
  wires:
  Hall/1 -> Bit concatenate/1(u)
  Bit concatenate/1(y) -> Data Type Conversion/1
  Data Type Conversion/1 -> Bias/1
  Bias/1 -> Scope/1, Direct Lookup Table (n-D)2/1
  Direct Lookup Table (n-D)2/1 -> S/1

== system PMSM_FOC_Traction/Motor_Control/Motor_Control_Funtion/FOC_Control_100us/FOC/Angle_set/Subsystem/Subsystem1 ==
  HFI_Angle : Inport
  Action Port : ActionPort  ActionPortLabel=if(u1 ==3)
  Out1 : Outport
  wires:
  HFI_Angle/1 -> Out1/1

== system PMSM_FOC_Traction/Motor_Control/Motor_Control_Funtion/FOC_Control_100us/FOC/Angle_set/Subsystem/Subsystem2 ==
  IPD_Angle : Inport
  Action Port : ActionPort  ActionPortLabel=elseif(u1 <3)
  Out1 : Outport
  wires:
  IPD_Angle/1 -> Out1/1

== system PMSM_FOC_Traction/Motor_Control/Motor_Control_Funtion/FOC_Control_100us/FOC/Flux_weakening /Subsystem/Flux_weak ==
  note: sqrt(Ud*Ud+Uq*Uq)<=Udc/sqrt(3)
  Vd : Inport
  Vq : Inport  Port=2
  id_input : Inport  Port=3
  Iq_input : Inport  Port=4
  Add1 : Sum  OutDataTypeStr=Inherit: Same as first input
  Constant : Constant  Value=pmsm.RatedVoltage/sqrt(3)  OutDataTypeStr=single  SampleTime=-1
  Fcn : Fcn  Expr=sqrt(u(1)^2+u(2)^2)
  ID_Control : Subsystem
  Mux : Mux  Inputs=2
  Sum1 : Sum  Inputs=|-+
  Id_ref : Outport
  iq_ref : Outport  Port=2
  wires:
  Constant/1 -> Sum1/2
  Sum1/1 -> ID_Control/1(Err)
  Mux/1 -> Fcn/1
  Fcn/1 -> Sum1/1
  Vq/1 -> Mux/2
  Iq_input/1 -> iq_ref/1
  id_input/1 -> Add1/1
  Vd/1 -> Mux/1
  Add1/1 -> Id_ref/1
  ID_Control/1(PI_Out) -> Add1/2

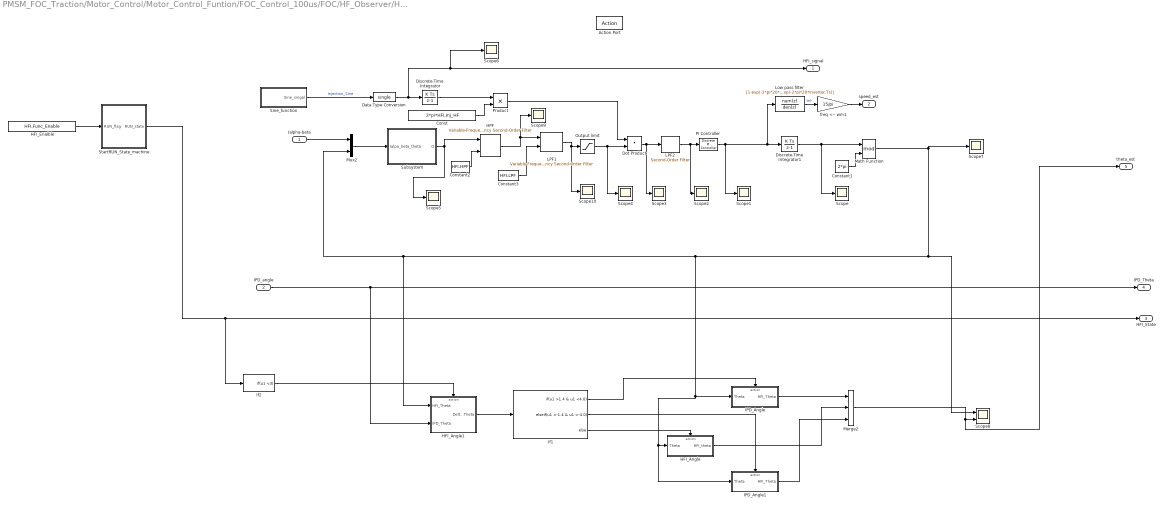
== system PMSM_FOC_Traction/Motor_Control/Motor_Control_Funtion/FOC_Control_100us/FOC/HF_Observer/HFI_Function/HFI ==
  Ialpha-beta : Inport
  IPD_angle : Inport  Port=2
  Action Port : ActionPort  ActionPortLabel=case [ 3 ]:
  Const : Constant  Value=2*pi*HFI.Inj_HF  OutDataTypeStr=single
  Constant1 : Constant  Value=2*pi  OutDataTypeStr=single
  Constant2 : Constant  Value=HFI.HPF  OutDataTypeStr=single
  Constant3 : Constant  Value=HFI.LPF  OutDataTypeStr=single
  Data Type Conversion : DataTypeConversion  OutDataTypeStr=single
  Discrete-Time Integrator : DiscreteIntegrator  SampleTime=-1  ICPrevOutput=DiscIntNeverNeededParam  ICPrevScaledInput=DiscIntNeverNeededParam
  Discrete-Time Integrator1 : DiscreteIntegrator  SampleTime=-1  ICPrevOutput=DiscIntNeverNeededParam  ICPrevScaledInput=DiscIntNeverNeededParam
  Dot Product : DotProduct  InputSameDT=on  OutDataTypeStr=Inherit: Inherit via internal rule
  HFI_Angle : Subsystem
  HFI_Angle1 : Subsystem
  HFI_Enalble : Constant  Value=HFI.Func_Enable  OutDataTypeStr=uint8
  HPF : eeGeneralControl/Variable-Frequency Second-Order Filter  FilterType=High-pass  fn=HFI.HPF  Zeta=single(0.707)  Ts=-1  A0=0  Ph0=0  f0=0  b0=0
      settings: SourceProductBaseCode=PS
  IPD_Angle : Subsystem
  IPD_Angle1 : Subsystem
  If1 : If  IfExpression=u1 >1.4 & u1 <4.0  ElseIfExpressions=u1 <-1.4 & u1 >-4.0
  If2 : If  IfExpression=u1 <3  ShowElse=off
  LPF1 : eeGeneralControl/Variable-Frequency Second-Order Filter  FilterType=Low-pass  fn=HFI.LPF  Zeta=single(0.707)  Ts=-1  A0=0  Ph0=0  f0=0  b0=0
      settings: SourceProductBaseCode=PS
  LPF2 : eeGeneralControl/Second-Order Filter  FilterType=Low-pass  fn=100  Zeta=single(0.707)  Ts=-1  A0=0  Ph0=0  f0=0  b0=0
      settings: SourceProductBaseCode=PS
  Low pass filter : DiscreteTransferFcn  Numerator=[1-exp(-2*pi*20*inverter.Ts)]  Denominator=[1 -exp(-2*pi*20*inverter.Ts)]
  Math Function : Math  Operator=mod  SignedPower=on  SaturateOnIntegerOverflow=on
  Merge2 : Merge  Inputs=3
  Mux2 : Mux  Inputs=2
  Output limit : Saturate
  PI Controller : powerlib_extras/Discrete  Control Blocks/Discrete PI Controller  Kp=HFI.PI_Kp  Ki=HFI.PI_Ki  Par_Limits=[100*2*pi -100*2*pi]  Init=0  Ts=-1
  Product : Product
  Scope{,1..7,9..10} (10 alike) : Scope
  Scope8 : Scope  NumInputPorts=2
  Sine_function : Subsystem
      settings: RTWSystemCode=Nonreusable function  RTWFcnNameOpts=Use subsystem name
  StartRUN_State_machine : Stateflow chart  TreatAsAtomicUnit=on
      settings: RTWSystemCode=Nonreusable function  RTWFcnNameOpts=Use subsystem name
  Subsystem : Subsystem
  freq <-- wm1 : Gain  Gain=15/pi
  HFI_signal : Outport
  speed_est : Outport  Port=2
  HFI_State : Outport  Port=3
  IPD_Theta : Outport  Port=4
  theta_est : Outport  Port=5
  wires:
  Mux2/1 -> Subsystem/1(Ialpa_beta_theta)
  Ialpha-beta/1 -> Mux2/1
  Subsystem/1(Q) -> HPF/1, Scope5/1
  freq <-- wm1/1 -> speed_est/1
  Discrete-Time Integrator1/1 -> Scope/1, Math Function/1
  LPF1/1 -> Scope10/1, Output limit/1
  LPF2/1 -> Scope2/1, PI Controller/1
  Low pass filter/1 -> freq <-- wm1/1  "we"
  HPF/1 -> LPF1/1, Scope9/1
  Discrete-Time Integrator/1 -> Product/1
  Product/1 -> Dot Product/1
  Dot Product/1 -> LPF2/1, Scope3/1
  Constant1/1 -> Math Function/2
  Output limit/1 -> Scope4/1, Dot Product/2
  Const/1 -> Product/2
  Sine_function/1(Sine_singal) -> Data Type Conversion/1  "Injection_Sine"
  Data Type Conversion/1 -> Scope6/1, HFI_signal/1, Discrete-Time Integrator/1
  HFI_Enalble/1 -> StartRUN_State_machine/1(RUN_flag)
  StartRUN_State_machine/1(RUN_state) -> If2/1, HFI_State/1
  IPD_angle/1 -> HFI_Angle1/2(IPD_Theta), IPD_Theta/1
  Math Function/1 -> IPD_Angle1/1(Theta), HFI_Angle/1(Theta), IPD_Angle/1(Theta), HFI_Angle1/1(HFI_Theta), Mux2/2, Scope8/1, Scope7/1
  PI Controller/1 -> Low pass filter/1, Discrete-Time Integrator1/1, Scope1/1
  If1/1 -> IPD_Angle/Action
  HFI_Angle/1(HFI_theta) -> Merge2/2
  If1/3 -> HFI_Angle/Action
  IPD_Angle/1(HFI_Theta) -> Merge2/1
  HFI_Angle1/1(Delta_Theta) -> If1/1
  If2/1 -> HFI_Angle1/Action
  Merge2/1 -> theta_est/1, Scope8/2
  If1/2 -> IPD_Angle1/Action
  IPD_Angle1/1(HFI_Theta) -> Merge2/3
  Constant2/1 -> HPF/2
  Constant3/1 -> LPF1/2

== system PMSM_FOC_Traction/Motor_Control/Motor_Control_Funtion/FOC_Control_100us/FOC/HF_Observer/HFI_Function/IPD ==
  Iabc : Inport  PortDimensions=3
  Action Port : ActionPort  ActionPortLabel=case [ 1 ]:
  7 : Fcn  Expr=u[1]*u[3]
  8 : Fcn  Expr=u[1]*u[2]
  Constant : Constant  Value=HFI.IPD_V
  Demux1 : Demux  Outputs=3
  HF_Angle : Subsystem
  Mux : Mux  Inputs=3
  Scope : Scope
  Sine_Cosine : Subsystem  TreatAsAtomicUnit=on
      settings: RTWSystemCode=Nonreusable function  RTWFcnNameOpts=Use subsystem name
  Theta_cacl : Subsystem
      settings: RTWSystemCode=Nonreusable function
  Ualpha : Outport
  Ubeta : Outport  Port=2
  Theta : Outport  Port=3
  wires:
  Sine_Cosine/1(Sin) -> Mux/2
  Sine_Cosine/2(Cos) -> Mux/3
  Constant/1 -> Mux/1
  Mux/1 -> 8/1, 7/1
  7/1 -> Ualpha/1
  8/1 -> Ubeta/1
  Iabc/1 -> Scope/1, Demux1/1  "Phase_CurrentABC"
  HF_Angle/1(Theta_V) -> Sine_Cosine/1(P)
  Demux1/3 -> Theta_cacl/3(Ic)
  Demux1/2 -> Theta_cacl/2(Ib)
  Theta_cacl/1(Theta) -> Theta/1
  Demux1/1 -> Theta_cacl/1(Ia)

== system PMSM_FOC_Traction/Motor_Control/Motor_Control_Funtion/FOC_Control_100us/FOC/HF_Observer/HFI_Function/NS ==
  Id : Inport
  Theta : Inport  Port=2
  Action Port : ActionPort  ActionPortLabel=case [ 2 ]:
  Abs : Abs
  Abs1 : Abs
  Data Type Conversion : DataTypeConversion
  Delay : Delay  DelayLength=1  InitialCondition=0
  Delay1 : Delay  DelayLength=1  InitialCondition=0
  HFI_Enalble : Constant  Value=HFI.Func_Enable  OutDataTypeStr=uint8
  Merge : Merge  Inputs=5
  Merge1 : Merge  Inputs=5
  NS_State_machine : Stateflow chart  TreatAsAtomicUnit=on
      settings: RTWSystemCode=Nonreusable function  RTWFcnNameOpts=Use subsystem name
  Scope1 : Scope  NumInputPorts=2
  Switch Case1 : SwitchCase  CaseConditions={1,2,3,4,5}  ShowDefaultCase=off
  Ud_inject_1 : Subsystem
  Ud_inject_2 : Subsystem
  Ud_inject_3 : Subsystem
  Ud_inject_4 : Subsystem
  Ud_inject_5 : Subsystem
  Ualpha : Outport
  Ubeta : Outport  Port=2
  IPD_Angle : Outport  Port=3
  Angle_RUN : Outport  Port=4
  wires:
  HFI_Enalble/1 -> NS_State_machine/1(NS_flag1)
  NS_State_machine/1(NS_state) -> Switch Case1/1
  Id/1 -> Ud_inject_2/1(Id), Ud_inject_4/1(Id)
  Merge/1 -> Scope1/1, Ualpha/1
  Ud_inject_2/1(Ualpha) -> Merge/1
  Ud_inject_4/1(Ualpha) -> Merge/2
  Merge1/1 -> Scope1/2, Ubeta/1
  Ud_inject_2/2(Ubeta) -> Merge1/1
  Ud_inject_4/2(Ubeta) -> Merge1/2
  Ud_inject_4/3(Id_out) -> Delay1/1
  Ud_inject_2/3(Id_out) -> Delay/1
  Ud_inject_1/1(Ualpha) -> Merge/3
  Ud_inject_1/2(Ubeta) -> Merge1/3
  Ud_inject_3/1(Ualpha) -> Merge/4
  Ud_inject_3/2(Ubeta) -> Merge1/4
  Switch Case1/1 -> Ud_inject_1/Action
  Switch Case1/2 -> Ud_inject_2/Action
  Theta/1 -> Ud_inject_4/2(Theta), Ud_inject_2/2(Theta), Ud_inject_1/1(Theta), Ud_inject_5/1(Theta), Ud_inject_3/1(Theta)
  Switch Case1/3 -> Ud_inject_3/Action
  Switch Case1/4 -> Ud_inject_4/Action
  Switch Case1/5 -> Ud_inject_5/Action
  Ud_inject_5/1(Ualpha) -> Merge/5
  Ud_inject_5/2(Ubeta) -> Merge1/5
  Abs/1 -> Ud_inject_5/2(Id1)
  Abs1/1 -> Ud_inject_5/3(Id2)
  Ud_inject_5/3(IPD_Angle) -> Data Type Conversion/1, IPD_Angle/1
  Delay/1 -> Abs/1
  Delay1/1 -> Abs1/1
  Data Type Conversion/1 -> Angle_RUN/1

== system PMSM_FOC_Traction/Motor_Control/Motor_Control_Funtion/Angle_Speed_100us/Flux_OBSERVER/equ3.12/integrator/RangeLimit/If Action Subsystem ==
  In1 : Inport  OutDataTypeStr=single
  Action Port : ActionPort  ActionPortLabel=elseif(u2)
  Constant : Constant  Value=2*pi  OutDataTypeStr=single  SampleTime=-1
  Sum : Sum  Inputs=|++  OutDataTypeStr=single
  Out1 : Outport  OutDataTypeStr=single
  wires:
  In1/1 -> Sum/1
  Constant/1 -> Sum/2
  Sum/1 -> Out1/1

== system PMSM_FOC_Traction/Motor_Control/Motor_Control_Funtion/Angle_Speed_100us/Flux_OBSERVER/equ3.12/integrator/RangeLimit/If Action Subsystem1 ==
  In1 : Inport  OutDataTypeStr=single
  Action Port : ActionPort  ActionPortLabel=if(u1)
  Constant : Constant  Value=2*pi  OutDataTypeStr=single  SampleTime=-1
  Sum : Sum  Inputs=|+-  OutDataTypeStr=single
  Out1 : Outport  OutDataTypeStr=single
  wires:
  In1/1 -> Sum/1
  Constant/1 -> Sum/2
  Sum/1 -> Out1/1

== system PMSM_FOC_Traction/Motor_Control/Motor_Control_Funtion/Angle_Speed_100us/Flux_OBSERVER/equ3.12/integrator/RangeLimit/If Action Subsystem2 ==
  In1 : Inport  OutDataTypeStr=single
  Action Port : ActionPort  ActionPortLabel=else
  Out1 : Outport  OutDataTypeStr=single
  wires:
  In1/1 -> Out1/1

== system PMSM_FOC_Traction/Motor_Control/Motor_Control_Funtion/Angle_Speed_100us/HIGH_SMO/QPLL/SpeedToTheta/RangeLimit/If Action Subsystem ==
  In1 : Inport
  Action Port : ActionPort  ActionPortLabel=elseif(u2)
  Constant : Constant  Value=2*pi  OutDataTypeStr=single  SampleTime=-1
  Sum : Sum  Inputs=|++
  Out1 : Outport
  wires:
  In1/1 -> Sum/1
  Constant/1 -> Sum/2
  Sum/1 -> Out1/1

== system PMSM_FOC_Traction/Motor_Control/Motor_Control_Funtion/Angle_Speed_100us/HIGH_SMO/QPLL/SpeedToTheta/RangeLimit/If Action Subsystem1 ==
  In1 : Inport
  Action Port : ActionPort  ActionPortLabel=if(u1)
  Constant : Constant  Value=2*pi  OutDataTypeStr=single  SampleTime=-1
  Sum : Sum  Inputs=|+-
  Out1 : Outport
  wires:
  In1/1 -> Sum/1
  Constant/1 -> Sum/2
  Sum/1 -> Out1/1

== system PMSM_FOC_Traction/Motor_Control/Motor_Control_Funtion/Angle_Speed_100us/HIGH_SMO/QPLL/SpeedToTheta/RangeLimit/If Action Subsystem2 ==
  In1 : Inport
  Action Port : ActionPort  ActionPortLabel=else
  Out1 : Outport
  wires:
  In1/1 -> Out1/1

== system PMSM_FOC_Traction/Motor_Control/Motor_Control_Funtion/Angle_Speed_100us/SpeedAndAngle/ACC_OMG/BLDC/Control/Commutation ==
  Hall : Inport
  Bias : Bias  Bias=-1
  Bit concatenate : Subsystem
  Data Type Conversion : DataTypeConversion
  Direct Lookup Table (n-D)2 : LookupNDDirect  InputsSelectThisObjectFromTable=Vector  Table=[0 0 0 1 1 0;0 1 1 0 0 0;0 1 0 0 0 1;1 0 0 0 1 0;1 0 1 0 0 0;0 0 0 1 0 1]  TableDataTypeStr=single
  Scope : Scope
  S : Outport  VectorParamsAs1DForOutWhenUnconnected=off
  wires:
  Hall/1 -> Bit concatenate/1(u)
  Bit concatenate/1(y) -> Data Type Conversion/1
  Direct Lookup Table (n-D)2/1 -> S/1
  Data Type Conversion/1 -> Bias/1
  Bias/1 -> Scope/1, Direct Lookup Table (n-D)2/1

== system PMSM_FOC_Traction/Motor_Control/Motor_Control_Funtion/Angle_Speed_100us/SpeedAndAngle/ACC_OMG/BLDC/Control/Speed_Control ==
  Err : Inport
  Action Port : ActionPort  ActionPortLabel=if(u1==3)
  Add : Sum
  Cons : Constant  Value=0  OutDataTypeStr=single
  Discrete-Time Integrator : DiscreteIntegrator  SampleTime=-1  ICPrevOutput=DiscIntNeverNeededParam  ICPrevScaledInput=DiscIntNeverNeededParam
  Ki : Constant  Value=17.72  OutDataTypeStr=single
  Kp : Constant  Value=0.7476  OutDataTypeStr=single
  Product : Product
  Product1 : Product
  Relational Operator1 : RelationalOperator  Operator===  OutDataTypeStr=boolean  RndMeth=Simplest
  Saturation : Saturate  UpperLimit=4200  LowerLimit=0
  Scope : Scope
  Switch : Switch  Criteria=u2 > Threshold
  Unit Delay3 : UnitDelay  SampleTime=-1  HasFrameUpgradeWarning=on
  PI_Out : Outport
  wires:
  Kp/1 -> Product/1
  Err/1 -> Switch/1, Product/2
  Switch/1 -> Product1/2
  Product1/1 -> Discrete-Time Integrator/1
  Product/1 -> Add/1
  Add/1 -> Relational Operator1/1, Saturation/1
  Saturation/1 -> Relational Operator1/2, PI_Out/1
  Discrete-Time Integrator/1 -> Add/2, Scope/1
  Relational Operator1/1 -> Unit Delay3/1
  Ki/1 -> Product1/1
  Unit Delay3/1 -> Switch/2
  Cons/1 -> Switch/3

== system PMSM_FOC_Traction/Motor_Control/Motor_Control_Funtion/Angle_Speed_100us/SpeedAndAngle/Subsystem/Subsystem1/Commutation/Bit concatenate ==
  u : Inport
  Gain : Gain  Gain=[4 2 1]  Multiplication=Matrix(K*u)
  Sum of Elements : Sum  Inputs=+
  y : Outport  VectorParamsAs1DForOutWhenUnconnected=off
  wires:
  u/1 -> Gain/1
  Gain/1 -> Sum of Elements/1
  Sum of Elements/1 -> y/1

== system PMSM_FOC_Traction/Motor_Control/Motor_Control_Funtion/FOC_Control_100us/FOC/Flux_weakening /Subsystem/Flux_weak/ID_Control ==
  Err : Inport
  Add : Sum
  Cons : Constant  Value=0  OutDataTypeStr=single
  Discrete-Time Integrator : DiscreteIntegrator  SampleTime=-1  ICPrevOutput=DiscIntNeverNeededParam  ICPrevScaledInput=DiscIntNeverNeededParam
  Ki : Constant  Value=ki  OutDataTypeStr=single
  Kp : Constant  Value=kp  OutDataTypeStr=single
  Product : Product
  Product1 : Product
  Relational Operator1 : RelationalOperator  Operator===  OutDataTypeStr=boolean  RndMeth=Simplest
  Saturation : Saturate  UpperLimit=Id_max  LowerLimit=Id_min
  Switch : Switch  Criteria=u2 > Threshold
  Unit Delay3 : UnitDelay  SampleTime=-1  HasFrameUpgradeWarning=on
  PI_Out : Outport
  wires:
  Kp/1 -> Product/1
  Err/1 -> Switch/1, Product/2
  Switch/1 -> Product1/2
  Product1/1 -> Discrete-Time Integrator/1
  Product/1 -> Add/1
  Add/1 -> Relational Operator1/1, Saturation/1
  Saturation/1 -> Relational Operator1/2, PI_Out/1
  Cons/1 -> Switch/3
  Discrete-Time Integrator/1 -> Add/2
  Relational Operator1/1 -> Unit Delay3/1
  Ki/1 -> Product1/1
  Unit Delay3/1 -> Switch/2

== system PMSM_FOC_Traction/Motor_Control/Motor_Control_Funtion/FOC_Control_100us/FOC/HF_Observer/HFI_Function/HFI/HFI_Angle ==
  Theta : Inport
  Action Port : ActionPort  ActionPortLabel=else
  HFI_theta : Outport
  wires:
  Theta/1 -> HFI_theta/1

== system PMSM_FOC_Traction/Motor_Control/Motor_Control_Funtion/FOC_Control_100us/FOC/HF_Observer/HFI_Function/HFI/HFI_Angle1 ==
  HFI_Theta : Inport
  IPD_Theta : Inport  Port=2
  Action Port : ActionPort  ActionPortLabel=if(u1 <3)
  Subtract : Sum  Inputs=+-
  Delta_Theta : Outport
  wires:
  HFI_Theta/1 -> Subtract/1
  IPD_Theta/1 -> Subtract/2
  Subtract/1 -> Delta_Theta/1

== system PMSM_FOC_Traction/Motor_Control/Motor_Control_Funtion/FOC_Control_100us/FOC/HF_Observer/HFI_Function/HFI/IPD_Angle ==
  Theta : Inport
  Action Port : ActionPort  ActionPortLabel=if(u1 >1.4 & u1 <4.0)
  Angle_calibration : Subsystem  TreatAsAtomicUnit=on
      settings: RTWSystemCode=Nonreusable function  RTWFcnNameOpts=Use subsystem name
  HFI_Theta : Outport
  wires:
  Theta/1 -> Angle_calibration/1(Angle_input)
  Angle_calibration/1(Angle_output) -> HFI_Theta/1

== system PMSM_FOC_Traction/Motor_Control/Motor_Control_Funtion/FOC_Control_100us/FOC/HF_Observer/HFI_Function/HFI/IPD_Angle1 ==
  Theta : Inport
  Action Port : ActionPort  ActionPortLabel=elseif(u1 <-1.4 & u1 >-4.0)
  Angle_calibration : Subsystem  TreatAsAtomicUnit=on
      settings: RTWSystemCode=Nonreusable function  RTWFcnNameOpts=Use subsystem name
  HFI_Theta : Outport
  wires:
  Theta/1 -> Angle_calibration/1(Angle_input)
  Angle_calibration/1(Angle_output) -> HFI_Theta/1

== system PMSM_FOC_Traction/Motor_Control/Motor_Control_Funtion/FOC_Control_100us/FOC/HF_Observer/HFI_Function/HFI/Sine_function ==
  A : Gain  Gain=HFI.Inj_HV
  Add : Sum
  Const1 : Constant  Value=2*pi*inverter.Ts*HFI.Inj_HF  OutDataTypeStr=single
  Const2 : Constant  Value=2*pi  OutDataTypeStr=single
  Const3 : Constant  Value=0  OutDataTypeStr=single
  Const4 : Constant  OutDataTypeStr=single
  Delay : Delay  DelayLength=1  InitialCondition=0
  Memory : Memory  InheritSampleTime=on
  Product1 : Product
  Relational Operator1 : RelationalOperator  Operator=<  OutDataTypeStr=boolean  RndMeth=Simplest
  Sine : Lookup_n-D  NumberOfTableDimensions=1  LookupTableObject=''  BreakpointsForDimension1=[0:2*pi/4095:2*pi]  BreakpointsForDimension1FirstPoint=10  BreakpointsForDimension2FirstPoint=10  BreakpointsForDimension1Spacing=12  BreakpointsForDimension2Spacing=12  IndexSearchMethod=Evenly spaced points  Table=Sine_table  InterpMethod=Flat  DiagnosticForOutOfRangeInput=Error  InternalRulePriority=Speed  RndMeth=Simplest  InputSameDT=on
  Switch : Switch  Criteria=u2 > Threshold
  Sine_singal : Outport
  wires:
  Switch/1 -> Product1/1
  Const3/1 -> Switch/3
  Relational Operator1/1 -> Switch/2
  Delay/1 -> Relational Operator1/1
  Const2/1 -> Relational Operator1/2
  Add/1 -> Memory/1, Delay/1
  Sine/1 -> A/1
  Product1/1 -> Sine/1, Add/2
  Memory/1 -> Product1/2
  Const1/1 -> Add/1
  Const4/1 -> Switch/1
  A/1 -> Sine_singal/1

== system PMSM_FOC_Traction/Motor_Control/Motor_Control_Funtion/FOC_Control_100us/FOC/HF_Observer/HFI_Function/HFI/Subsystem ==
  Ialpa_beta_theta : Inport
  Add2 : Sum  Inputs=-+  OutDataTypeStr=Inherit: Same as first input
  Demux : Demux  Outputs=2
  Demux1 : Demux  Outputs=2
  Produc3t : Product  RndMeth=Simplest  OutDataTypeStr=Inherit: Same as first input
  Product4 : Product  RndMeth=Simplest  OutDataTypeStr=Inherit: Same as first input
  Sine_Cosine : Subsystem
      settings: RTWSystemCode=Nonreusable function  RTWFcnNameOpts=Use subsystem name
  Q : Outport  VectorParamsAs1DForOutWhenUnconnected=off
  wires:
  Add2/1 -> Q/1
  Sine_Cosine/2(Cos) -> Product4/2
  Produc3t/1 -> Add2/1
  Sine_Cosine/1(Sin) -> Produc3t/2
  Product4/1 -> Add2/2
  Demux/1 -> Produc3t/1
  Demux/2 -> Product4/1
  Demux1/1 -> Demux/1
  Demux1/2 -> Sine_Cosine/1(P)
  Ialpa_beta_theta/1 -> Demux1/1

== system PMSM_FOC_Traction/Motor_Control/Motor_Control_Funtion/FOC_Control_100us/FOC/HF_Observer/HFI_Function/IPD/HF_Angle ==
  Add : Sum
  Const1 : Constant  Value=2*pi*inverter.Ts*HFI.IPD_F  OutDataTypeStr=single
  Const2 : Constant  Value=2*pi  OutDataTypeStr=single
  Const3 : Constant  Value=0  OutDataTypeStr=single
  Const4 : Constant  OutDataTypeStr=single
  Delay : Delay  DelayLength=1  InitialCondition=0
  Memory : Memory  InheritSampleTime=on
  Product1 : Product
  Relational Operator1 : RelationalOperator  Operator=<  OutDataTypeStr=boolean  RndMeth=Simplest
  Switch : Switch  Criteria=u2 > Threshold
  Theta_V : Outport
  wires:
  Switch/1 -> Product1/1
  Delay/1 -> Relational Operator1/1
  Const2/1 -> Relational Operator1/2
  Const3/1 -> Switch/3
  Relational Operator1/1 -> Switch/2
  Const1/1 -> Add/1
  Memory/1 -> Product1/2
  Add/1 -> Memory/1, Delay/1
  Product1/1 -> Theta_V/1, Add/2
  Const4/1 -> Switch/1

== system PMSM_FOC_Traction/Motor_Control/Motor_Control_Funtion/FOC_Control_100us/FOC/HF_Observer/HFI_Function/IPD/Sine_Cosine ==
  note: Sine Cosine Coefficients
  P : Inport
  Cosine : Lookup_n-D  NumberOfTableDimensions=1  LookupTableObject=''  BreakpointsForDimension1=[0:2*pi/4095:2*pi]  BreakpointsForDimension1FirstPoint=10  BreakpointsForDimension2FirstPoint=10  BreakpointsForDimension1Spacing=12  BreakpointsForDimension2Spacing=12  IndexSearchMethod=Evenly spaced points  Table=Cosine_table  InterpMethod=Flat  DiagnosticForOutOfRangeInput=Error  InternalRulePriority=Speed  RndMeth=Simplest  InputSameDT=on
  Scope : Scope  NumInputPorts=2
  Sine : Lookup_n-D  NumberOfTableDimensions=1  LookupTableObject=''  BreakpointsForDimension1=[0:2*pi/4095:2*pi]  BreakpointsForDimension1FirstPoint=10  BreakpointsForDimension2FirstPoint=10  BreakpointsForDimension1Spacing=12  BreakpointsForDimension2Spacing=12  IndexSearchMethod=Evenly spaced points  Table=Sine_table  InterpMethod=Flat  DiagnosticForOutOfRangeInput=Error  InternalRulePriority=Speed  RndMeth=Simplest  InputSameDT=on
  Sin : Outport  VectorParamsAs1DForOutWhenUnconnected=off
  Cos : Outport  Port=2  VectorParamsAs1DForOutWhenUnconnected=off
  wires:
  P/1 -> Cosine/1, Sine/1  "position"
  Sine/1 -> Scope/1, Sin/1
  Cosine/1 -> Scope/2, Cos/1
